simulink model "Simulation_3221"  (R2023a)
settings: Solver=VariableStepAuto  StartTime=0.0  StopTime=600  RelTol=1e-3
undefined symbols (not defined in the file or in its folder): Ion, Lithium
libraries: spsSeriesRLCBranchLib x14, simulink x11, spsBatteryLib x10, spsControlledCurrentSourceLib x10, spsCurrentMeasurementLib x7, spsVoltageMeasurementLib x7, spsControlledVoltageSourceLib x3, spspowerguiLib x1
(part 1 of 3)
settings Model: Creator=40485811  LastModifiedBy=40485811

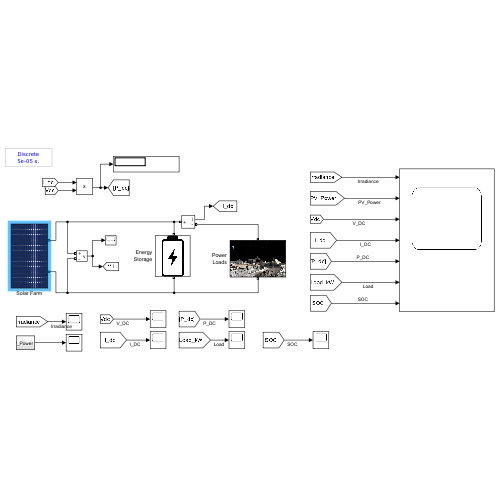
[thumbnail: Simulink's stored preview of the top-level diagram]
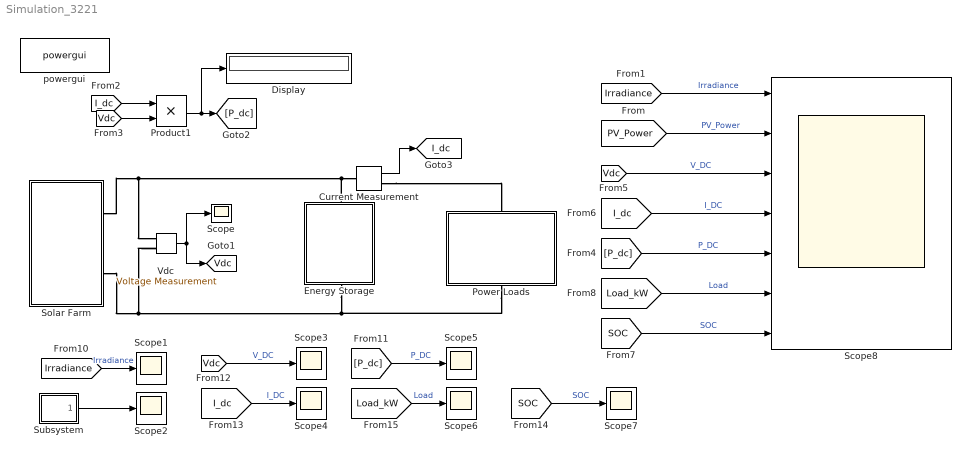
== system Simulation_3221 ==
  Current Measurement : spsCurrentMeasurementLib/Current Measurement  PhasorSimulation=off  OutputType=Complex  PSBequivalent=0
  Display : Display
  Energy Storage : Subsystem
      settings: PortSchema="{\"entries\":[{\"content\":{\"sides\":[{\"content\":{},\"type\":\"ConnectorPlacement.EquallySpacedRectSide\",\"uuid\":\"19301019-6073-4742-9acf-f42e8adc5c9e\"},{\"content\":{\"side\":\"RIGHT\"},\"type\":\"ConnectorPlacement.EquallySpacedRectSide\",\"uuid\":\"e7e8b761-1860-4e60-96a0-e09456fe9b7d\"},{\"content\":{\"connectorIds\":[\"LConn1\"],\"side\":\"TOP\"},\"type\":\"ConnectorPlacement.EquallySpacedRectSide\",\"uuid\":\"9a2c7ab2-e8b2-40d2-a24e-d56c39a325f7\"},{\"content\":{\"connectorIds\":[\"RConn1\"],\"side\":\"BOTTOM\"},\"type\":\"ConnectorPlacement.EquallySpacedRectSide\",\"uuid\":\"a05fc25a-9576-4133-8247-40976c625624\"}]},\"type\":\"ConnectorPlacement.EquallySpacedConnector\",\"uuid\":\"018c4af4-b2b6-48b3-8fd0-4a05f6dfe868\"}],\"packageUris\":[\"http://schema.mathworks.com/mf0/Connector/R2020b\"],\"version\":\"1.0\"}"
      mask Display: image('\\napier-mail.napier.ac.uk\students\School of Engineering and the Built Environment\User Data\40485811\My Profile\Downloads\battery-icon-13.png'); % Use "Edit Image" on toolstrip to change.
  Power Loads : Subsystem
      mask Display: image('\\napier-mail.napier.ac.uk\students\School of Engineering and the Built Environment\User Data\40485811\My Profile\Downloads\Untitled.png'); % Use "Edit Image" on toolstrip to change.
  Product1 : Product
  Scope{,1..7} (8 alike) : Scope
  Scope8 : Scope  NumInputPorts=7
  Solar Farm : Subsystem
      mask Display: image('\\napier-mail.napier.ac.uk\students\School of Engineering and the Built Environment\User Data\40485811\My Profile\Downloads\istockphoto-1441533310-612x612.jpg'); % Use "Edit Image" on toolstrip to change.
  Subsystem : Subsystem
  "Vdc " : spsVoltageMeasurementLib/Voltage Measurement  Tag=PoWeRsYsTeMmEaSuReMeNt  PhasorSimulation=off  OutputType=Magnitude  PSBequivalent=0
  powergui : spspowerguiLib/powergui  Priority=1  SimulationMode=Discrete  SampleTime=5e-5  frequency=60  Iterations=50  frequencyindice=0  Pbase=100e6  ErrMax=1e-4  UnitsV=kV  UnitsW=MW  buscounter=0  FunctionMessages=off  echomessages=off  EnableUseOfTLC=off  CurrentSourceSwitches=off  DisableSnubberDevices=off  DisableRonSwitches=off  DisableVfSwitches=off  DisplayEquations=off  AutomaticDiscreteSolvers=off  SolverType=Tustin  Interpol=off  ExternalGateDelay=off  methode=off  Ts=0  x0status=blocks  SPID=off  SwTol=0  HookPort=off  NonlinearTolerance=1e-4  nMaxIteration=100  ContinueOnMaxIteration=off  RestoreLinks=warning  ResistiveCurrentMeasurement=off  Frange=[0:2:500]  Ylog=off  Xlog=on  ShowGrid=off  save=off  variable=ZData  structure=0  ZoomFFT=on  StartTime=0.0  cycles=1  DisplayStyle=1  fundamental=60  FreqAxis=off  MaxFrequency=1000  frequencyindicesteady=1  RmsSteady=1  display=off
  tag scope: I_dc=global, Vdc=global
  wires:
  [I_dc] -> Product1/1
  [Vdc] -> Product1/2
  Product1/1 -> Display/1, [P_dc]
  [Irradiance] -> Scope8/1  "Irradiance"
  [PV_Power] -> Scope8/2  "PV_Power"
  [Vdc] -> Scope8/3  "V_DC"
  [I_dc] -> Scope8/4  "I_DC"
  [P_dc] -> Scope8/5  "P_DC"
  [SOC] -> Scope8/7  "SOC"
  [Load_kW] -> Scope8/6  "Load"
  "Vdc "/1 -> Scope/1, [Vdc]
  Current Measurement/1 -> [I_dc]
  [SOC] -> Scope7/1  "SOC"
  [Load_kW] -> Scope6/1  "Load"
  [P_dc] -> Scope5/1  "P_DC"
  [I_dc] -> Scope4/1  "I_DC"
  [Vdc] -> Scope3/1  "V_DC"
  [Irradiance] -> Scope1/1  "Irradiance"
  Subsystem/1(PV_Power) -> Scope2/1
  connections:
  Current Measurement/LConn1 -- Solar Farm/RConn1 -- "Vdc "/LConn1 -- Energy Storage/LConn1
  Power Loads/RConn1 -- "Vdc "/LConn2 -- Solar Farm/RConn2 -- Energy Storage/RConn1
  Current Measurement/RConn1 -- Power Loads/LConn1

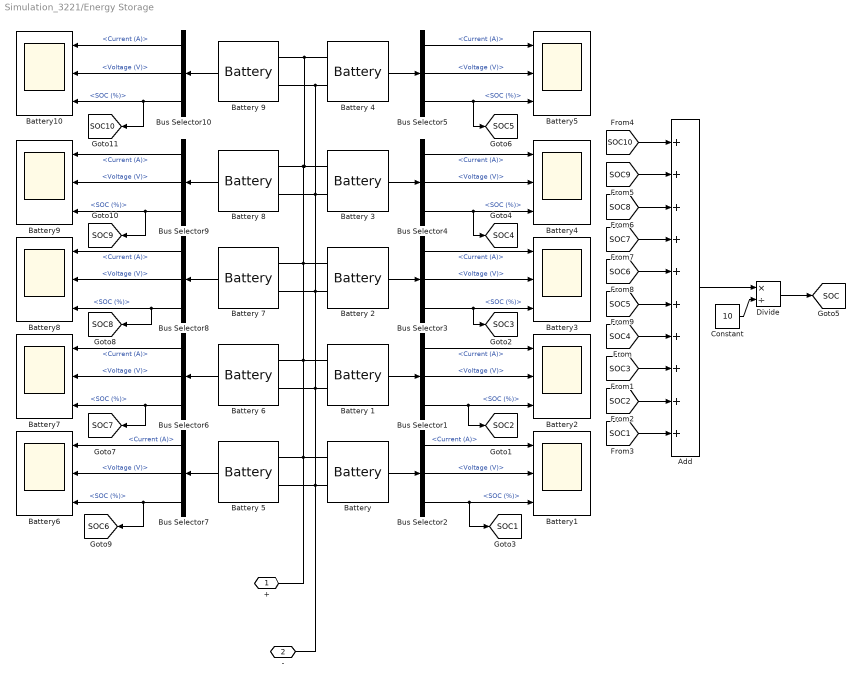
== system Simulation_3221/Energy Storage ==
  Add : Sum  Inputs=++++++++++
  Battery {,1..9} (10 alike) : spsBatteryLib/Battery  BatType=Lithium-Ion  ShowTempParam=off  ThermalPreset=no  ShowAgeParam=off  NomV=11  NomQ=20000  SOC=50  Batt_Tr=0.1  PresetModel=on  MaxQ=20000  MinV=8.25  FullV=12.8039  Dis_rate=8695.6522  R=5.5e-06  Normal_OP=18086.9565  expZone="[11.88424      982.6087]"  current=[6.5 13 32.5]  Units=Time  Tci=20  NomT=20  T2=-30  MaxQ2=4.8  FullV2=7.1  Normal_OP2=5.655  expZone2="[6.58           1]"  Rca=0.6  ti=2000  Dp=0  Neq0=0  Tsim=1e6  Ta1=25  Qeol=5.4*0.9  Reol=0.013333*1.2  Char_age=[2.3478, 3]  Dis_age=[2.3478, 10]  N1=1500  N2=10500  N3=1000  N4=1400  Ta2=45  N5=950
  Battery{1..10} (10 alike) : Scope  NumInputPorts=3
  Bus Selector{1..10} (10 alike) : BusSelector  OutputSignals=Current (A),Voltage (V),SOC (%)
  Constant : Constant  Value=10
  Divide : Product  Inputs=*/
  + : PMIOPort  Side=Left
  - : PMIOPort  Port=2  Side=Right
  tag scope: SOC10=global, SOC1=global, SOC2=global, SOC3=global, SOC4=global, SOC5=global, SOC6=global, SOC7=global, SOC8=global, SOC9=global, SOC=global
  wires:
  Battery 1/1 -> Bus Selector1/1
  Bus Selector4/2 -> Battery4/2  "<Voltage (V)>"
  Bus Selector1/1 -> Battery2/1  "<Current (A)>"
  Bus Selector2/1 -> Battery1/1  "<Current (A)>"
  Bus Selector3/3 -> [SOC3], Battery3/3  "<SOC (%)>"
  Bus Selector2/2 -> Battery1/2  "<Voltage (V)>"
  "Battery "/1 -> Bus Selector2/1
  Bus Selector2/3 -> Battery1/3, [SOC1]  "<SOC (%)>"
  Bus Selector4/1 -> Battery4/1  "<Current (A)>"
  Bus Selector3/1 -> Battery3/1  "<Current (A)>"
  Bus Selector3/2 -> Battery3/2  "<Voltage (V)>"
  Bus Selector4/3 -> [SOC4], Battery4/3  "<SOC (%)>"
  Bus Selector1/2 -> Battery2/2  "<Voltage (V)>"
  Bus Selector1/3 -> [SOC2], Battery2/3  "<SOC (%)>"
  [SOC4] -> Add/7
  [SOC1] -> Add/10
  [SOC3] -> Add/8
  [SOC2] -> Add/9
  Add/1 -> Divide/1
  Constant/1 -> Divide/2
  Divide/1 -> [SOC]
  Battery 3/1 -> Bus Selector4/1
  Battery 2/1 -> Bus Selector3/1
  Bus Selector5/3 -> [SOC5], Battery5/3  "<SOC (%)>"
  Battery 4/1 -> Bus Selector5/1
  Bus Selector5/1 -> Battery5/1  "<Current (A)>"
  Bus Selector5/2 -> Battery5/2  "<Voltage (V)>"
  Battery 9/1 -> Bus Selector10/1
  Bus Selector10/2 -> Battery10/2  "<Voltage (V)>"
  Battery 7/1 -> Bus Selector8/1
  Battery 6/1 -> Bus Selector6/1
  Bus Selector9/2 -> Battery9/2  "<Voltage (V)>"
  Bus Selector9/3 -> [SOC9], Battery9/3  "<SOC (%)>"
  Battery 8/1 -> Bus Selector9/1
  Bus Selector7/2 -> Battery6/2  "<Voltage (V)>"
  Bus Selector7/1 -> Battery6/1  "<Current (A)>"
  Bus Selector6/2 -> Battery7/2  "<Voltage (V)>"
  Bus Selector6/3 -> [SOC7], Battery7/3  "<SOC (%)>"
  Battery 5/1 -> Bus Selector7/1
  Bus Selector8/1 -> Battery8/1  "<Current (A)>"
  Bus Selector8/3 -> [SOC8], Battery8/3  "<SOC (%)>"
  Bus Selector10/3 -> [SOC10], Battery10/3  "<SOC (%)>"
  Bus Selector8/2 -> Battery8/2  "<Voltage (V)>"
  Bus Selector6/1 -> Battery7/1  "<Current (A)>"
  Bus Selector7/3 -> Battery6/3, [SOC6]  "<SOC (%)>"
  Bus Selector9/1 -> Battery9/1  "<Current (A)>"
  [SOC5] -> Add/6
  [SOC6] -> Add/5
  [SOC7] -> Add/4
  [SOC8] -> Add/3
  [SOC9] -> Add/2
  [SOC10] -> Add/1
  Bus Selector10/1 -> Battery10/1  "<Current (A)>"
  connections:
  Battery 9/LConn2 -- "Battery "/LConn2 -- -/RConn1 -- Battery 5/LConn2 -- Battery 1/LConn2 -- Battery 6/LConn2 -- Battery 2/LConn2 -- Battery 7/LConn2 -- Battery 3/LConn2 -- Battery 8/LConn2 -- Battery 4/LConn2
  Battery 9/LConn1 -- +/RConn1 -- "Battery "/LConn1 -- Battery 5/LConn1 -- Battery 1/LConn1 -- Battery 6/LConn1 -- Battery 2/LConn1 -- Battery 7/LConn1 -- Battery 8/LConn1 -- Battery 3/LConn1 -- Battery 4/LConn1

== system Simulation_3221/Power Loads ==
  Add Block : Sum  Inputs=+++
  Constant Loads : Subsystem
  Controlled Current Source block : spsControlledCurrentSourceLib/Controlled Current Source  Initialize=on  Source_Type=AC  Amplitude=0  Phase=0  Frequency=0  Measurements=None
  Divide : Product  Inputs=*/
  Industrial Loads : Subsystem
  Variable Loads : Subsystem
  - : PMIOPort  Side=Left
  + : PMIOPort  Port=2  Side=Right
  tag scope: Load_kW=global
  wires:
  [Vdc] -> Divide/2  "Grid Voltage"
  Add Block/1 -> [Load_kW], Divide/1
  Divide/1 -> Controlled Current Source block/1
  Constant Loads/1(Out1) -> Add Block/1
  Variable Loads/1(Out1) -> Add Block/2
  Industrial Loads/1(Out1) -> Add Block/3
  connections:
  Controlled Current Source block/RConn1 -- +/RConn1
  -/RConn1 -- Controlled Current Source block/LConn1
